simulink model "validation models"  (R2018a)
settings: Solver=VariableStepAuto  StartTime=0.0  StopTime=15  RelTol=1e-3
settings Model: Creator=Acer  LastModifiedBy=Acer

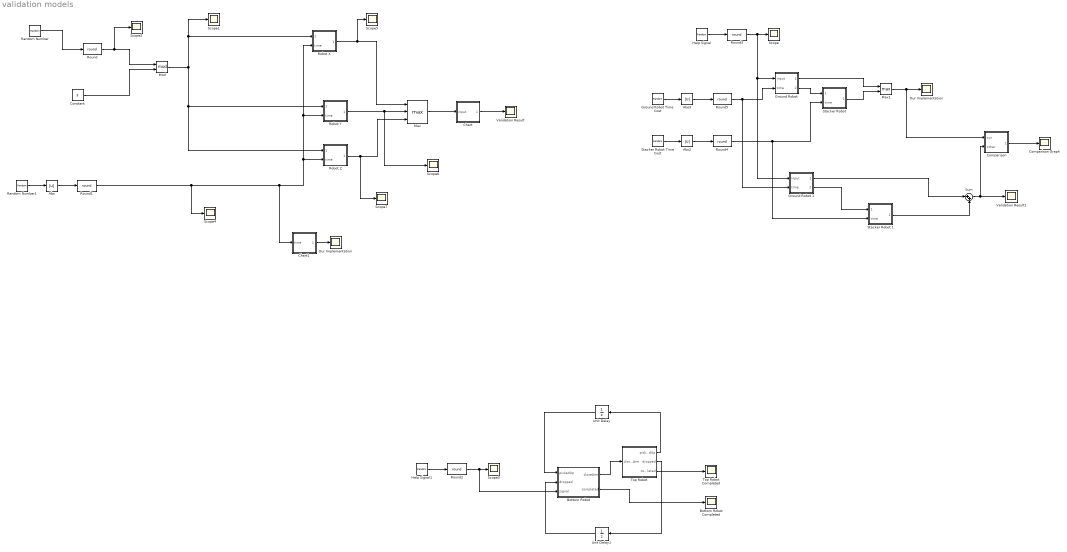
== system validation models ==
  Abs : Abs
  Abs2 : Abs
  Abs3 : Abs
  Bottom Robot : Stateflow chart  TreatAsAtomicUnit=on
  Bottom Robot Completed : Scope
  Chart : Stateflow chart  TreatAsAtomicUnit=on
  Chart1 : Stateflow chart  TreatAsAtomicUnit=on
  Comparison : Stateflow chart  TreatAsAtomicUnit=on
  "Comparison Graph " : Scope
  Constant : Constant  Value=3  OutDataTypeStr=double
  "Ground Robot " : Stateflow chart  TreatAsAtomicUnit=on
  Ground Robot 1 : Stateflow chart  TreatAsAtomicUnit=on
  Ground Robot Time Cost : RandomNumber  Mean=4  SampleTime=1
  Help Signal : UniformRandomNumber  Minimum=0  SampleTime=1
  Help Signal1 : UniformRandomNumber  Minimum=0  SampleTime=1
  Max : MinMax  Function=max  Inputs=3
  Max1 : MinMax  Function=max  Inputs=2
  Mod : Math  Operator=mod  SaturateOnIntegerOverflow=on
  Our Implementation : Scope
  "Our Implementation " : Scope
  Random Number : RandomNumber  Mean=2  Variance=3  Seed=11  SampleTime=1
  Random Number1 : RandomNumber  Mean=4  Seed=3  SampleTime=1
  Robot X : Stateflow chart  TreatAsAtomicUnit=on
  "Robot Y " : Stateflow chart  TreatAsAtomicUnit=on
  Robot Z : Stateflow chart  TreatAsAtomicUnit=on
  Round{,1..5} (6 alike) : Rounding  Operator=round
  Scope{,1..7} (8 alike) : Scope
  "Stacker Robot " : Stateflow chart  TreatAsAtomicUnit=on
  Stacker Robot 1 : Stateflow chart  TreatAsAtomicUnit=on
  "Stacker Robot Time Cost " : RandomNumber  Mean=4  Seed=1  SampleTime=1
  Sum : Sum  Inputs=|++
  Top Robot : Stateflow chart  TreatAsAtomicUnit=on
  Top Robot Completed : Scope
  Unit Delay : UnitDelay
  Unit Delay1 : UnitDelay
  Validation Result : Scope
  Validation Result1 : Scope
  wires:
  Abs/1 -> Round1/1
  Max/1 -> Chart/1(input)
  Round/1 -> Scope2/1, Mod/1
  Random Number/1 -> Round/1
  Robot Z/1(output) -> Scope7/1, Max/3
  "Robot Y "/1(output) -> Scope6/1, Max/2
  Chart/1(output) -> Validation Result/1
  Constant/1 -> Mod/2
  Mod/1 -> Robot Z/1(taskID), "Robot Y "/1(taskID), Scope1/1, Robot X/1(taskID)
  Random Number1/1 -> Abs/1
  Round1/1 -> Scope4/1, Chart1/1(time), Robot Z/2(time), Robot X/2(time), "Robot Y "/2(time)
  Robot X/1(output) -> Scope5/1, Max/1
  Chart1/1(output) -> "Our Implementation "/1
  Ground Robot 1/1(output) -> Sum/1
  Abs2/1 -> Round4/1
  "Stacker Robot Time Cost "/1 -> Abs2/1
  Round4/1 -> Stacker Robot 1/2(time), "Stacker Robot "/2(time)
  "Stacker Robot "/1(output) -> Max1/2
  Ground Robot Time Cost/1 -> Abs3/1
  "Ground Robot "/2(needHelp) -> "Stacker Robot "/1(needHelp)
  Sum/1 -> Comparison/2(other), Validation Result1/1
  Round3/1 -> Scope/1, Ground Robot 1/1(input), "Ground Robot "/1(input)
  "Ground Robot "/1(output) -> Max1/1
  Comparison/1(output) -> "Comparison Graph "/1
  Stacker Robot 1/1(output) -> Sum/2
  Ground Robot 1/2(needHelp) -> Stacker Robot 1/1(needHelp)
  Abs3/1 -> Round5/1
  Round5/1 -> Ground Robot 1/2(time), "Ground Robot "/2(time)
  Max1/1 -> Comparison/1(our), Our Implementation/1
  Help Signal/1 -> Round3/1
  Top Robot/1(pickedUp) -> Unit Delay/1
  Bottom Robot/1(closeArm) -> Top Robot/1(closeArm)
  Top Robot/2(dropped) -> Unit Delay1/1
  Bottom Robot/2(completed) -> Bottom Robot Completed/1
  Top Robot/3(completed) -> Top Robot Completed/1
  Help Signal1/1 -> Round2/1
  Round2/1 -> Bottom Robot/3(signal), Scope3/1
  Unit Delay/1 -> Bottom Robot/1(pickedUp)
  Unit Delay1/1 -> Bottom Robot/2(dropped)

== stateflow chart validation models/Robot Z ==
  state INIT
    during: oldTime = 0
    during: output = 1
  state BUSY
    during: output = 1
    during: oldTime = oldTime - 1
  state FASTFORWARD
  (default) -> INIT
  BUSY -> INIT [order 2] : [oldTime == 0]
  INIT -> BUSY : [taskID == 2]{oldTime = time}
  BUSY -> FASTFORWARD [order 1] : [taskID == 0]{output = oldTime}
  FASTFORWARD -> BUSY : {oldTime = time}
  data: taskID input double; output output double; time input double; oldTime local double

== stateflow chart validation models/Robot Y  ==
  state INIT
    during: oldTime = 0
    during: output = 1
  state BUSY
    during: output = 1
    during: oldTime = oldTime - 1
  state FASTFORWARD
  (default) -> INIT
  BUSY -> INIT [order 2] : [oldTime == 0]
  INIT -> BUSY : [taskID == 1]{oldTime = time}
  BUSY -> FASTFORWARD [order 1] : [taskID == 0]{output = oldTime}
  FASTFORWARD -> BUSY : {oldTime = time}
  data: taskID input double; output output double; time input double; oldTime local double

== stateflow chart validation models/Robot X ==
  state INIT
    during: oldTime = 0
    during: output = 1
  state BUSY
    during: output = 1
    during: oldTime = oldTime - 1
  state FASTFORWARD
  (default) -> INIT
  BUSY -> INIT [order 2] : [oldTime == 0]
  INIT -> BUSY : [taskID == 0]{oldTime = time}
  BUSY -> FASTFORWARD [order 1] : [taskID == 0]{output = oldTime}
  FASTFORWARD -> BUSY : {oldTime = time}
  data: taskID input double; output output double; time input double; oldTime local double

== stateflow chart validation models/Chart ==
  state IDLE
    entry: output = 0
    during: output = output + input
  (default) -> IDLE
  data: input input double; output output double

== stateflow chart validation models/Chart1 ==
  state INIT
    entry: x = 0
    entry: y = 0
    entry: z = 0
    entry: output = 0
    during: x = 0
    during: y = 0
    during: z = 0
    during: output = output + 1
  state Z
    during: z = z - 1
    during: output = output + 1
  state XZ
    during: x = x - 1
    during: z = z - 1
    during: output = output + 1
  state YZ
    during: y = y - 1
    during: z = z - 1
    during: output = output + 1
  state Y
    during: y = y - 1
    during: output = output + 1
  state X
    during: x = x - 1
    during: output = output + 1
  state XY
    during: x = x - 1
    during: y = y - 1
    during: output = output + 1
  state XXYZ
    during: x = x - 1
    during: y = y - 1
    during: z = z - 1
  state XYZ
    during: x = x - 1
    during: y = y - 1
    during: z = z - 1
    during: output = output + 1
  state XYZZ
    during: x = x - 1
    during: y = y - 1
    during: z = z - 1
  state XYYZ
    during: x = x - 1
    during: y = y - 1
    during: z = z - 1
  (default) -> INIT
  Z -> INIT [order 2] : [z <= 0 && time == 0]{z = 0; output = output + 1}
  Y -> INIT [order 1] : [y <= 0 && time == 0]{y = 0; output = output + 1}
  YZ -> Z [order 2] : [y <= 0 && time == 0]{y = 0; output = output + 1}
  Z -> X [order 1] : [z <= 0 && time > 0]{z = 0; x = time; output = output + 1}
  X -> INIT [order 2] : [x <= 0 && time == 0]{output = output + 1}
  INIT -> X : [time > 0]{x = time; output = output + 1}
  Z -> XZ [order 3] : [z > 0 && time > 0]{x = time; output = output + 1}
  XZ -> Z [order 3] : [x <= 0]{x = 0; output = output + 1}
  YZ -> XZ [order 4] : [time > 0 && y <= 0]{x = time; output = output + 1}
  XZ -> X [order 2] : [z <= 0]{z = 0; output = output + 1}
  Y -> X [order 2] : [y <= 0 && time > 0]{x = time; output = output + 1}
  YZ -> Y [order 3] : [z <= 0 && time == 0]{z = 0; output = output + 1}
  X -> X [order 3] : [x == 0 && time > 0]{x = time; output = output + 1}
  XZ -> XYZ [order 1] : [time > 0 && x > 0 && z > 0]{x = x - 1; z = z - 1; output = output + 1}
  XYZ -> XZ [order 2] : [y <= 0]{y = 0; output = output + 1}
  YZ -> XYZ [order 1] : [time > 0 && y > 0 && z > 0]{x = time; output = output + 1}
  XYZ -> YZ [order 4] : [x <= 0 && y > 0 && z > 0 && time == 0]{x = 0; output = output + 1}
  Y -> XY [order 3] : [y > 0 && time > 0]{x = time; output = output + 1}
  XY -> Y [order 4] : [y > 0 && x <= 0 && time == 0]{x = 0; output = output + 1}
  XY -> X [order 1] : [y <= 0 && time == 0]{y = 0; output = output + 1}
  X -> XY [order 1] : [time > 0 && x > 0]{x = x - 1; y = time; output = output + 1}
  XY -> XYZ [order 2] : [time > 0 && x > 0 && y > 0]{x = x - 1; y = y - 1; z =  time; output = output + 1}
  XYZ -> XXYZ [order 5] : [time > 0 && x <= y && x < z]{output = output + x; x = time}
  XYZ -> XY [order 1] : [z <= 0 && time == 0 && x > 0 && y > 0]{z = 0; output = output + 1}
  XXYZ -> XYZ
  XYZ -> XYZ [order 3] : [z <= 0 && x > 0 && y > 0 && time > 0]{z = time}
  XY -> XY [order 3] : [y <= 0 && x > 0 && time > 0]{y = time; output = output + 1}
  XYZZ -> XYZ
  XYZ -> XYZZ [order 7] : [time > 0 && z < y && z < x]{output = output + z; z = time}
  XYYZ -> XYZ
  XYZ -> XYYZ [order 6] : [x > y && y <= z && time > 0]{output = output + y; y = time}
  data: time input; output output; x local; y local; z local

== stateflow chart validation models/Ground Robot  ==
  state INIT
    entry: needHelp = 0
    entry: output = 0
    during: needHelp = 0
    during: output = time
  state HELP
    during: needHelp = 1
    during: output = time
  (default) -> INIT
  HELP -> INIT : [input == 0]{needHelp = 0; output = 0}
  INIT -> HELP : [input == 1]{needHelp = 1; output = time}
  data: output output double; input input double; needHelp output double; time input double

== stateflow chart validation models/Stacker Robot  ==
  state INIT
    entry: output = 0
    during: output = 0
  state HELP
    during: output = time
  (default) -> INIT
  INIT -> HELP : [needHelp == 1]{output = time}
  HELP -> INIT : [needHelp == 0]{output = 0}
  data: output output double; needHelp input double; time input double

== stateflow chart validation models/Bottom Robot ==
  state INIT
    during: time = time + 1
    during: closeArm = 0
  state DROP
  state TRAVEL
    during: closeArm = 1
    during: time = time + 1
  state IDLE
  (default) -> INIT : {time = 0; closeArm = 0; completed = 0}
  DROP -> INIT : [dropped == 1]{completed = completed + 1}
  INIT -> IDLE : [time > 3 && signal == 1]{closeArm = 1}
  TRAVEL -> DROP : [time > 5]{closeArm = 0; time = 0}
  IDLE -> TRAVEL : [pickedUp == 1]{time = 0}
  data: time local; closeArm output; completed output; pickedUp input; dropped input; signal input

== stateflow chart validation models/Ground Robot 1 ==
  state INIT
    entry: needHelp = 0
    entry: output = 0
    during: needHelp = 0
    during: output = time
  state HELP
    during: needHelp = 1
    during: output = time
  (default) -> INIT
  HELP -> INIT : [input == 0]{needHelp = 0; output = 0}
  INIT -> HELP : [input == 1]{needHelp = 1; output = time}
  data: output output double; input input double; needHelp output double; time input double

== stateflow chart validation models/Stacker Robot 1 ==
  state INIT
    entry: output = 0
    during: output = 0
  state HELP
    during: output = time
  (default) -> INIT
  INIT -> HELP : [needHelp == 1]{output = time}
  HELP -> INIT : [needHelp == 0]{output = 0}
  data: output output double; needHelp input double; time input double

== stateflow chart validation models/Comparison ==
  state INIT
    entry: output = 0
    during: output = 0
  state OTHER
    during: output = -1
  state OUR
    during: output = 1
  (default) -> INIT
  OTHER -> INIT [order 1] : [our == other]{output = 0}
  OUR -> INIT [order 2] : [our == other]{output = 0}
  INIT -> OUR : [our < other]{output = 1}
  OUR -> OTHER [order 1] : [our > other]{output = -1}
  OTHER -> OUR [order 2] : [our < other]{output = 1}
  data: our input double; other input double; output output double

== stateflow chart validation models/Top Robot ==
  state INIT
    during: time = time + 1
    during: pickedUp = 0
  state DROP
    during: time = time + 1
  state IDLE
    during: time = time + 1
  state TRAVEL
  (default) -> INIT : {pickedUp = 0; time = 0; dropped = 0; completed = 0}
  DROP -> INIT : [time > 1]{dropped = 1; completed = completed + 1}
  INIT -> IDLE : [closeArm == 1]
  TRAVEL -> DROP : [closeArm == 0]{time = 0}
  IDLE -> TRAVEL : [time > 1]{pickedUp = 1; time = 0}
  data: pickedUp output; time local; dropped output; completed output; closeArm input
